simulink model "sumfilter_u8_8"  (R2023a)
settings: Solver=FixedStepDiscrete  StartTime=0.0  StopTime=2  RelTol=1e-3
values from neighbouring files (symbols this model uses):
  R = 752    [setup.m]
undefined symbols (not defined in the file or in its folder): gray
libraries: hdlsllib x15, visionhdlio x5, visionsources x2, simulink_extras x2
Description:
  | Sobel Edge Detection Using the MATLAB(R) Function Block
  | This example shows how to use HDL Coder(TM) to check,
  | generate, and verify HDL code for a Sobel Edge Detection
  | block built using the MATLAB Function block.
settings Model: Creator=The MathWorks, Inc.  LastModifiedBy=njv3788
settings SolverCC: AlgebraicLoopSolver=TrustRegion
settings DataIOCC: LimitDataPoints=on  SaveFormat=Array  SignalLogging=off  ReturnWorkspaceOutputs=off
settings OptimizationCC: BlockReduction=off  ConditionallyExecuteInputs=off  DefaultParameterBehavior=Inlined  ExpressionDepthLimit=2147483647  InitFltsAndDblsToZero=on  EfficientMapNaN2IntZero=off  LifeSpan=inf
settings DebuggingCC: AlgebraicLoopMsg=error  SaveWithParameterizedLinksMsg=none  UnderspecifiedInitializationDetection=Classic  MergeDetectMultiDrivingBlocksExec=none  SignalResolutionControl=TryResolveAllWithWarning  MultiTaskDSMMsg=warning  MultiTaskCondExecSysMsg=none  SingleTaskRateTransMsg=error  IntegerOverflowMsg=none  ParameterPrecisionLossMsg=none  FcnCallInpInsideContextMsg=warning  UnconnectedInputMsg=warning  UnconnectedOutputMsg=warning  UnconnectedLineMsg=warning  AllowSymbolicDim=off  StateNameClashWarn=warning  StrictBusMsg=ErrorOnBusTreatedAsVector  SFUnexpectedBacktrackingDiag=warning  SFNoUnconditionalDefaultTransitionDiag=warning  SFExecutionAtInitializationDiag=none  IntegerSaturationMsg=none  ArithmeticOperatorsInVariantConditions=warning
settings HardwareCC: ProdBitPerPointer=32  ProdBitPerSizeT=32  ProdBitPerPtrDiffT=32  ProdLargestAtomicFloat=None  ProdIntDivRoundTo=Undefined  ProdEndianess=Unspecified  ProdWordSize=32  ProdHWDeviceType=ASIC/FPGA  TargetHWDeviceType=32-bit Generic  ProdEqTarget=off
settings ModelReferenceCC: EnableRefExpFcnMdlSchedulingChecks=on  PropagateSignalLabelsOutOfModel=off
settings SFSimCC: SimUseLocalCustomCode=off  CustomCodeUndefinedFunction=UseInterfaceOnly
settings RTWCC: RTWUseLocalCustomCode=off  DLArmComputeVersion=19.05
settings CodeAppCC: StateflowObjectComments=on
settings GRTTargetCC: TargetFcnLib=ansi_tfl_tmw.mat  TargetLangStandard=C89/C90 (ANSI)  CombineOutputUpdateFcns=off  GRTInterface=on
settings ConfigComp: CovMetricSettings=dw  CovSaveCumulativeToWorkspaceVar=on  CovSaveSingleToWorkspaceVar=on  CovExternalEMLEnable=off

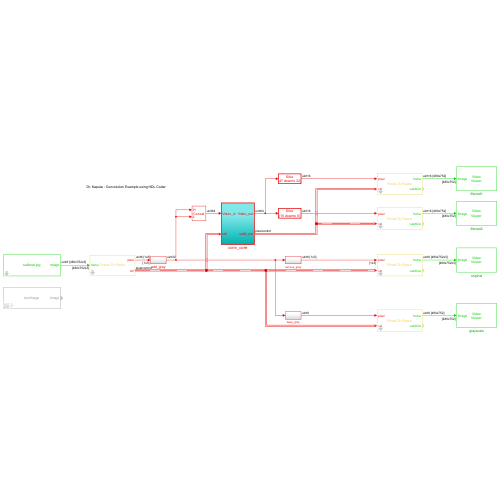
[thumbnail: Simulink's stored preview of the top-level diagram]
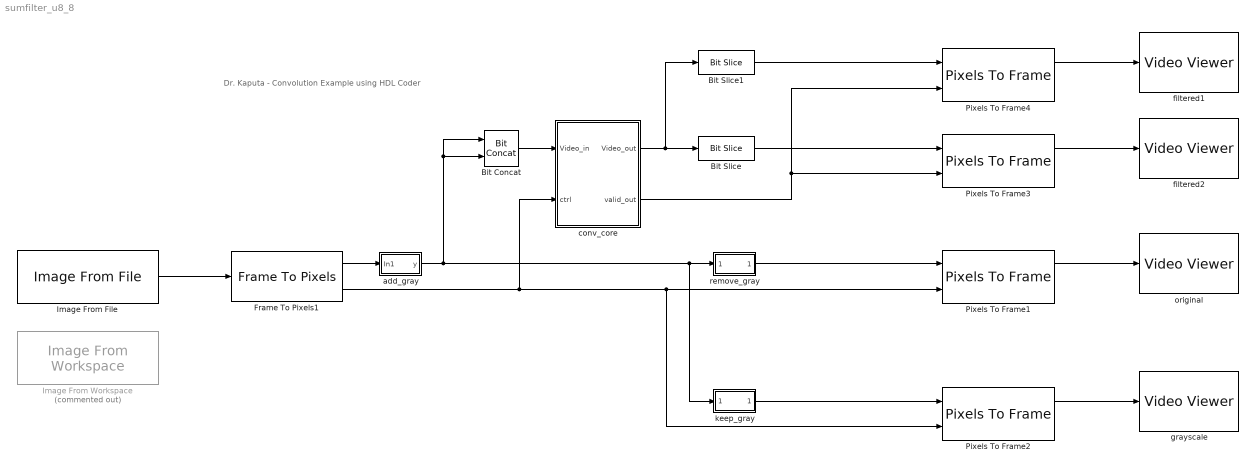
== system sumfilter_u8_8 ==
  note: Dr. Kaputa - Convolution Example using HDL Coder
  Bit Concat : hdlsllib/Logic and Bit Operations/Bit Concat  numInputs=2
  Bit Slice : hdlsllib/Logic and Bit Operations/Bit Slice  lidx=15  ridx=0
  Bit Slice1 : hdlsllib/Logic and Bit Operations/Bit Slice  lidx=47  ridx=32
  Frame To Pixels1 : visionhdlio/Frame To Pixels  NumComponents=3  NumPixels=1  VideoFormat=Custom  ActivePixelsPerLine=R  ActiveVideoLines=C  TotalPixelsPerLine=R  TotalVideoLines=C  StartingActiveLine=1  FrontPorch=0  SampleTime=0  VideoFormatCache=Custom  ActivePixelsPerLineCache=R  ActiveVideoLinesCache=C  TotalPixelsPerLineCache=R  TotalVideoLinesCache=C  StartingActiveLineCache=1  FrontPorchCache=0
  Image From File : visionsources/Image From File  Tag=vipblks_nd  FileName=sailboat.jpg  Ts=1  imagePorts=One multidimensional signal  OutPortLabels=R|G|B  ImageDataType=Inherit from input image  sdImageDataType=uint(8)  Signed=on  WordLength=16  FractionLengthMode=User-defined  FractionLength=15
  Image From Workspace : visionsources/Image From Workspace  Tag=vipblks_nd  Commented=on  ImageValue=testImage  Ts=1  imagePorts=One multidimensional signal  OutPortLabels=R|G|B  ImageDataType=Inherit from 'Value'  Signed=on  WordLength=16  sdImageDataType=sfix(16)  FractionLengthMode=User-defined  FractionLength=15
  Pixels To Frame1 : visionhdlio/Pixels To Frame  NumComponents=3  NumPixels=1  VideoFormat=Custom  ActivePixelsPerLine=R  ActiveVideoLines=C  TotalPixelsPerLine=R  TotalVideoLines=C  VideoFormatCache=Custom  ActivePixelsPerLineCache=R  ActiveVideoLinesCache=C  TotalPixelsPerLineCache=R  TotalVideoLinesCache=C
  Pixels To Frame2 : visionhdlio/Pixels To Frame  NumComponents=1  NumPixels=1  VideoFormat=Custom  ActivePixelsPerLine=R  ActiveVideoLines=C  TotalPixelsPerLine=R  TotalVideoLines=C  VideoFormatCache=Custom  ActivePixelsPerLineCache=R  ActiveVideoLinesCache=C  TotalPixelsPerLineCache=R  TotalVideoLinesCache=C
  Pixels To Frame3 : visionhdlio/Pixels To Frame  NumComponents=1  NumPixels=1  VideoFormat=Custom  ActivePixelsPerLine=R  ActiveVideoLines=C  TotalPixelsPerLine=R  TotalVideoLines=C  VideoFormatCache=Custom  ActivePixelsPerLineCache=R  ActiveVideoLinesCache=C  TotalPixelsPerLineCache=R  TotalVideoLinesCache=C
  Pixels To Frame4 : visionhdlio/Pixels To Frame  NumComponents=1  NumPixels=1  VideoFormat=Custom  ActivePixelsPerLine=R  ActiveVideoLines=C  TotalPixelsPerLine=R  TotalVideoLines=C  VideoFormatCache=Custom  ActivePixelsPerLineCache=R  ActiveVideoLinesCache=C  TotalPixelsPerLineCache=R  TotalVideoLinesCache=C
  add_gray : Subsystem
  conv_core : Subsystem  TreatAsAtomicUnit=on
  filtered1 : VideoViewer  colormapValue=gray(256)  FigPos=[154 856 646 566]
  filtered2 : VideoViewer  colormapValue=gray(256)  FigPos=[802 855 533 568]
  grayscale : VideoViewer  FigPos=[2195 901 1097 520]
  keep_gray : Subsystem
  original : VideoViewer  FigPos=[2068 836 1280 622]
  remove_gray : Subsystem
  wires:
  Pixels To Frame1/1 -> original/1
  Frame To Pixels1/2 -> conv_core/2(ctrl), Pixels To Frame1/2, Pixels To Frame2/2
  remove_gray/1(RGBVector) -> Pixels To Frame1/1
  Frame To Pixels1/1 -> add_gray/1(In1)
  add_gray/1(y) -> Bit Concat/2, Bit Concat/1, keep_gray/1(RGB), remove_gray/1(RGB)
  Pixels To Frame2/1 -> grayscale/1
  keep_gray/1(RGBVector) -> Pixels To Frame2/1
  Pixels To Frame3/1 -> filtered2/1
  Bit Concat/1 -> conv_core/1(Video_in)
  Pixels To Frame4/1 -> filtered1/1
  conv_core/2(valid_out) -> Pixels To Frame4/2, Pixels To Frame3/2
  conv_core/1(Video_out) -> Bit Slice1/1, Bit Slice/1
  Image From File/1 -> Frame To Pixels1/1
  Bit Slice1/1 -> Pixels To Frame4/1
  Bit Slice/1 -> Pixels To Frame3/1

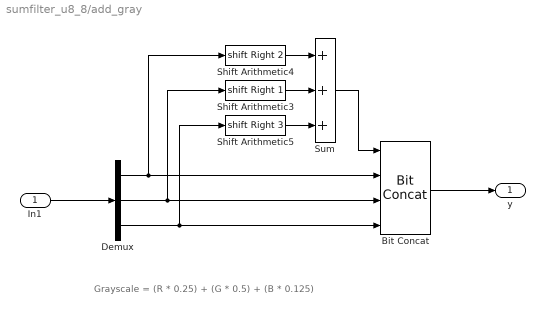
== system sumfilter_u8_8/add_gray ==
  note: Grayscale = (R * 0.25) + (G * 0.5) + (B * 0.125)
  In1 : Inport
  Bit Concat : hdlsllib/Logic and Bit Operations/Bit Concat  numInputs=4
  Demux : Demux  Outputs=3
  Shift Arithmetic3 : ArithShift  BitShiftNumber=1  BitShiftDirection=Right
  Shift Arithmetic4 : ArithShift  BitShiftNumber=2  BitShiftDirection=Right
  Shift Arithmetic5 : ArithShift  BitShiftNumber=3  BitShiftDirection=Right
  Sum : Sum  Inputs=+++  OutDataTypeStr=uint8
  y : Outport
  wires:
  Bit Concat/1 -> y/1
  In1/1 -> Demux/1
  Demux/2 -> Shift Arithmetic3/1, Bit Concat/3
  Demux/1 -> Shift Arithmetic4/1, Bit Concat/2
  Demux/3 -> Shift Arithmetic5/1, Bit Concat/4
  Sum/1 -> Bit Concat/1
  Shift Arithmetic4/1 -> Sum/1
  Shift Arithmetic3/1 -> Sum/2
  Shift Arithmetic5/1 -> Sum/3

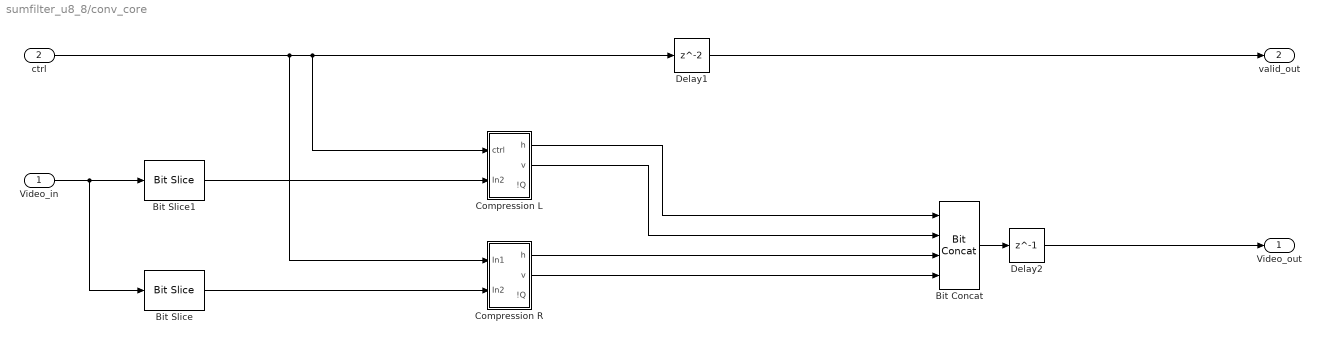
== system sumfilter_u8_8/conv_core ==
  Video_in : Inport
  ctrl : Inport  Port=2
  Bit Concat : hdlsllib/Logic and Bit Operations/Bit Concat  numInputs=4
  Bit Slice : hdlsllib/Logic and Bit Operations/Bit Slice  lidx=31  ridx=24
  Bit Slice1 : hdlsllib/Logic and Bit Operations/Bit Slice  lidx=63  ridx=56
  Compression L : Subsystem
  Compression R : Subsystem
  Delay1 : Delay  InitialCondition=0
  Delay2 : Delay  DelayLength=1  InitialCondition=0
  Video_out : Outport  VectorParamsAs1DForOutWhenUnconnected=off
  valid_out : Outport  Port=2  VectorParamsAs1DForOutWhenUnconnected=off
  wires:
  Delay1/1 -> valid_out/1
  Delay2/1 -> Video_out/1
  Bit Concat/1 -> Delay2/1
  Video_in/1 -> Bit Slice/1, Bit Slice1/1
  Bit Slice/1 -> Compression R/2(In2)
  Compression L/2(v) -> Bit Concat/2
  Compression L/1(h) -> Bit Concat/1
  ctrl/1 -> Compression R/1(In1), Compression L/1(ctrl), Delay1/1
  Bit Slice1/1 -> Compression L/2(In2)
  Compression R/1(h) -> Bit Concat/3
  Compression R/2(v) -> Bit Concat/4

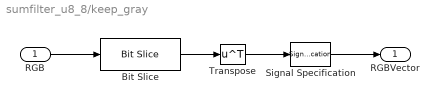
== system sumfilter_u8_8/keep_gray ==
  RGB : Inport
  Bit Slice : hdlsllib/Logic and Bit Operations/Bit Slice  lidx=31  ridx=24
  Signal Specification : SignalSpecification
  Transpose : Math  Operator=transpose  SignedPower=on
  RGBVector : Outport  VectorParamsAs1DForOutWhenUnconnected=off
  wires:
  RGB/1 -> Bit Slice/1
  Transpose/1 -> Signal Specification/1
  Signal Specification/1 -> RGBVector/1
  Bit Slice/1 -> Transpose/1

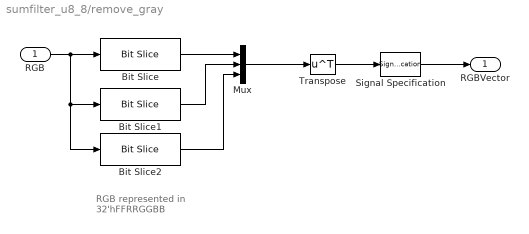
== system sumfilter_u8_8/remove_gray ==
  note: RGB represented in
      | 32'hFFRRGGBB
  RGB : Inport
  Bit Slice : hdlsllib/Logic and Bit Operations/Bit Slice  lidx=23  ridx=16
  Bit Slice1 : hdlsllib/Logic and Bit Operations/Bit Slice  lidx=15  ridx=8
  Bit Slice2 : hdlsllib/Logic and Bit Operations/Bit Slice  lidx=7  ridx=0
  Mux : Mux  Inputs=3
  Signal Specification : SignalSpecification
  Transpose : Math  Operator=transpose  SignedPower=on
  RGBVector : Outport  VectorParamsAs1DForOutWhenUnconnected=off
  wires:
  Signal Specification/1 -> RGBVector/1
  Transpose/1 -> Signal Specification/1
  RGB/1 -> Bit Slice/1, Bit Slice1/1, Bit Slice2/1
  Bit Slice1/1 -> Mux/2
  Bit Slice2/1 -> Mux/3
  Bit Slice/1 -> Mux/1
  Mux/1 -> Transpose/1

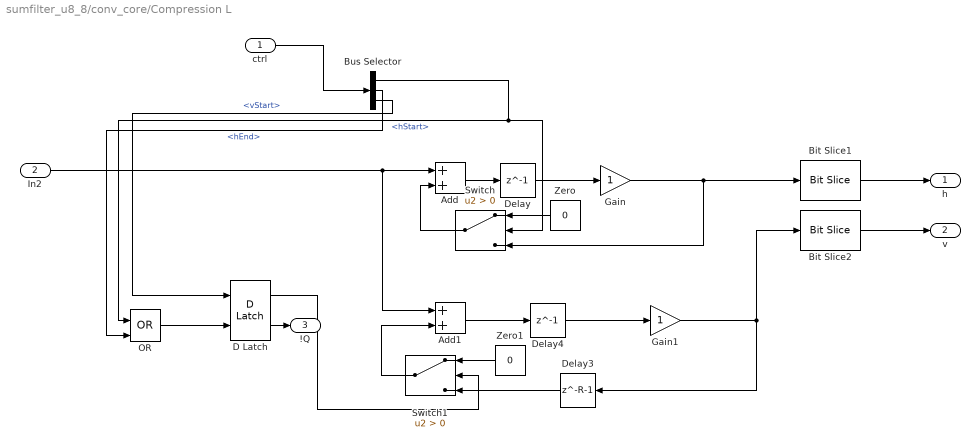
== system sumfilter_u8_8/conv_core/Compression L ==
  ctrl : Inport
  In2 : Inport  Port=2
  Add : Sum  AccumDataTypeStr=uint32
  Add1 : Sum  AccumDataTypeStr=uint32
  Bit Slice1 : hdlsllib/Logic and Bit Operations/Bit Slice  lidx=17  ridx=2
  Bit Slice2 : hdlsllib/Logic and Bit Operations/Bit Slice  lidx=16  ridx=1
  Bus Selector : BusSelector  OutputSignals=hStart,hEnd,vStart
  D Latch : simulink_extras/Flip Flops/D Latch
  Delay : Delay  DelayLength=1
  Delay3 : Delay  DelayLength=R-1
  Delay4 : Delay  DelayLength=1
  Gain : Gain  OutDataTypeStr=uint32
  Gain1 : Gain  OutDataTypeStr=uint32
  OR : Logic  Operator=OR  IconShape=distinctive  AllPortsSameDT=off  OutDataTypeStr=boolean
  Switch : Switch  Criteria=u2 > Threshold  OutDataTypeStr=uint32  SaturateOnIntegerOverflow=off  InputSameDT=off
  Switch1 : Switch  Criteria=u2 > Threshold  OutDataTypeStr=uint32  SaturateOnIntegerOverflow=off  InputSameDT=off
  Zero : Constant  Value=0  OutDataTypeStr=uint32
  Zero1 : Constant  Value=0  OutDataTypeStr=uint32
  h : Outport
  v : Outport  Port=2
  !Q : Outport  Port=3
  wires:
  OR/1 -> D Latch/2
  Add/1 -> Delay/1
  D Latch/2 -> !Q/1
  Bit Slice1/1 -> h/1
  Bus Selector/1 -> OR/1, Switch/2  "<hStart>"
  Add1/1 -> Delay4/1
  Zero/1 -> Switch/1
  Delay/1 -> Gain/1
  In2/1 -> Add1/1, Add/1
  Delay4/1 -> Gain1/1
  Switch/1 -> Add/2
  Zero1/1 -> Switch1/1
  Bit Slice2/1 -> v/1
  Bus Selector/3 -> D Latch/1  "<vStart>"
  Bus Selector/2 -> OR/2  "<hEnd>"
  Gain/1 -> Switch/3, Bit Slice1/1
  Delay3/1 -> Switch1/3
  D Latch/1 -> Switch1/2
  Gain1/1 -> Delay3/1, Bit Slice2/1
  Switch1/1 -> Add1/2
  ctrl/1 -> Bus Selector/1

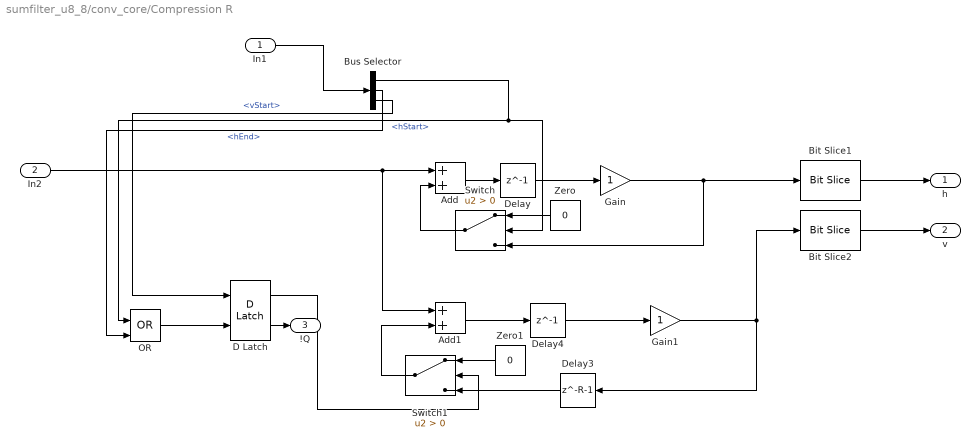
== system sumfilter_u8_8/conv_core/Compression R ==
  In1 : Inport
  In2 : Inport  Port=2
  Add : Sum  AccumDataTypeStr=uint32
  Add1 : Sum  AccumDataTypeStr=uint32
  Bit Slice1 : hdlsllib/Logic and Bit Operations/Bit Slice  lidx=17  ridx=2
  Bit Slice2 : hdlsllib/Logic and Bit Operations/Bit Slice  lidx=16  ridx=1
  Bus Selector : BusSelector  OutputSignals=hStart,hEnd,vStart
  D Latch : simulink_extras/Flip Flops/D Latch
  Delay : Delay  DelayLength=1
  Delay3 : Delay  DelayLength=R-1
  Delay4 : Delay  DelayLength=1
  Gain : Gain  OutDataTypeStr=uint32
  Gain1 : Gain  OutDataTypeStr=uint32
  OR : Logic  Operator=OR  IconShape=distinctive  AllPortsSameDT=off  OutDataTypeStr=boolean
  Switch : Switch  Criteria=u2 > Threshold  OutDataTypeStr=uint32  SaturateOnIntegerOverflow=off  InputSameDT=off
  Switch1 : Switch  Criteria=u2 > Threshold  OutDataTypeStr=uint32  SaturateOnIntegerOverflow=off  InputSameDT=off
  Zero : Constant  Value=0  OutDataTypeStr=uint32
  Zero1 : Constant  Value=0  OutDataTypeStr=uint32
  h : Outport
  v : Outport  Port=2
  !Q : Outport  Port=3
  wires:
  OR/1 -> D Latch/2
  Add/1 -> Delay/1
  D Latch/2 -> !Q/1
  Bit Slice1/1 -> h/1
  Bus Selector/1 -> OR/1, Switch/2  "<hStart>"
  Add1/1 -> Delay4/1
  Zero/1 -> Switch/1
  Delay/1 -> Gain/1
  In2/1 -> Add1/1, Add/1
  Delay4/1 -> Gain1/1
  Switch/1 -> Add/2
  Zero1/1 -> Switch1/1
  Bit Slice2/1 -> v/1
  Bus Selector/3 -> D Latch/1  "<vStart>"
  Bus Selector/2 -> OR/2  "<hEnd>"
  Gain/1 -> Switch/3, Bit Slice1/1
  Delay3/1 -> Switch1/3
  D Latch/1 -> Switch1/2
  Gain1/1 -> Delay3/1, Bit Slice2/1
  Switch1/1 -> Add1/2
  In1/1 -> Bus Selector/1
